simulink model "SIMEX"  (R2019a)
settings: Solver=ode4  StartTime=0.0  StopTime=SIMTIME  FixedStep=T  RelTol=1e-3
values from neighbouring files (symbols this model uses):
  A1 = pi*((d1^2)/4)    (= 7.06858347058e-06)    [SIMEX_load.m]
  A2 = pi*((d2^2)/4)    (= 3.14159265359e-06)    [SIMEX_load.m]
  Be = 1300e6    (= 1300000000)    [SIMEX_load.m]
  Cd = 0.6    [SIMEX_load.m]
  Cv = Q0/((Umax-Ud)*sqrt(p0))    [SIMEX_load.m]
  p1 = 200e5    (= 20000000)    [SIMEX_load.m]
  RHO = 860    [SIMEX_load.m]
  TAU = 1/(2*pi*fb)    (= 0.0318309886184)    [SIMEX_load.m]
  Ud = 2    [SIMEX_load.m]
  V = 2e-3    (= 0.002)    [SIMEX_load.m]
undefined symbols (not defined in the file or in its folder): sgn
settings Model: Creator=handroos  LastModifiedBy=handroos

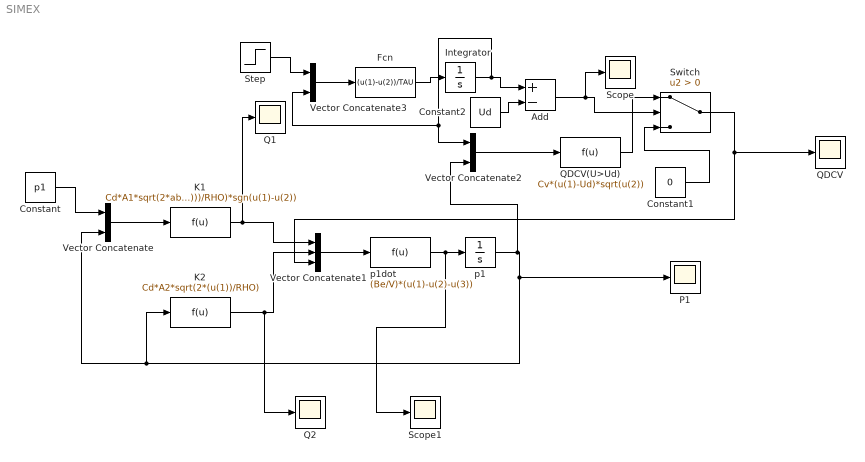
== system SIMEX ==
  Add : Sum  Inputs=+-
  Constant : Constant  Value=p1
  Constant1 : Constant  Value=0
  Constant2 : Constant  Value=Ud
  Fcn : Fcn  Expr=(u(1)-u(2))/TAU
  Integrator : Integrator
  K1 : Fcn  Expr=Cd*A1*sqrt(2*abs((u(1)-u(2)))/RHO)*sgn(u(1)-u(2))
  K2 : Fcn  Expr=Cd*A2*sqrt(2*(u(1))/RHO)
  P1 : Scope
  Q1 : Scope
  Q2 : Scope
  QDCV : Scope
  QDCV(U>Ud) : Fcn  Expr=Cv*(u(1)-Ud)*sqrt(u(2))
  Scope : Scope
  Scope1 : Scope
  Step : Step  Time=2  Before=2.5  After=4  SampleTime=0
  Switch : Switch  Criteria=u2 > Threshold
  Vector Concatenate : Concatenate
  Vector Concatenate1 : Concatenate  NumInputs=3
  Vector Concatenate2 : Concatenate
  Vector Concatenate3 : Concatenate
  p1 : Integrator  InitialCondition=100e5  LimitOutput=on  UpperSaturationLimit=1000e5  LowerSaturationLimit=0
  "p1dot " : Fcn  Expr=(Be/V)*(u(1)-u(2)-u(3))
  wires:
  Vector Concatenate/1 -> K1/1
  Constant/1 -> Vector Concatenate/1
  K1/1 -> Q1/1, Vector Concatenate1/1
  K2/1 -> Q2/1, Vector Concatenate1/2
  Vector Concatenate1/1 -> "p1dot "/1
  "p1dot "/1 -> Scope1/1, p1/1
  p1/1 -> Vector Concatenate2/2, P1/1, Vector Concatenate/2, K2/1
  Vector Concatenate2/1 -> QDCV(U>Ud)/1
  QDCV(U>Ud)/1 -> Switch/1
  Constant1/1 -> Switch/3
  Constant2/1 -> Add/2
  Add/1 -> Scope/1, Switch/2
  Switch/1 -> QDCV/1, Vector Concatenate1/3
  Fcn/1 -> Integrator/1
  Integrator/1 -> Vector Concatenate2/1, Vector Concatenate3/2, Add/1
  Vector Concatenate3/1 -> Fcn/1
  Step/1 -> Vector Concatenate3/1
